simulink model "Circuit3_v3"  (R2020b)
settings: Solver=ode4  StartTime=0.0  StopTime=SIMTIME  FixedStep=step  RelTol=1e-3
values from neighbouring files (symbols this model uses):
  Be1 = 1300e6    (= 1300000000)    [Circut3_values.m]
  Be_p = 1300e6    (= 1300000000)    [Circut3_values.m]
  BeA = 1200e6    (= 1200000000)    [Circuit2_values.m]    (also in Circut3_values.m = 1300000000)
  BeB = 1500e6    (= 1500000000)    [Circuit2_values.m]    (also in Circut3_values.m = 1300000000)
  C_cv = (70/60000)/sqrt(5e5)    [Circut3_values.m]
  C_o = (1/60000)/sqrt(5e5)    [Circut3_values.m]
  C_v_valve = 1.16e-8    (= 1.16e-08)    [Circut3_values.m]
  g = 9.81    [Circut3_values.m]
  Jm = 3.6e-3    (= 0.0036)    [Circut3_values.m]
  Kp = (1.e-3)/(10e5)    (= 1e-09)    [Circuit1_load.m]    (also in Circuit2_values.m; Circut3_values.m)
  ml = 500    [Circut3_values.m]
  mw = 100    [Circut3_values.m]
  nm = 0.93    [Circut3_values.m]
  p0 = 1.e5    (= 100000)    [Circuit1_load.m]    (also in Circut3_values.m = 200000)
  p10 = 73e5    (= 7300000)    [Circut3_values.m]
  pA0 = 1e5    (= 100000)    [Circuit2_values.m]    (also in Circut3_values.m = 7300000)
  pB0 = 1e5    (= 100000)    [Circuit2_values.m]    (also in Circut3_values.m = 700000)
  pref = 180e5    (= 18000000)    [Circuit1_load.m]    (also in Circuit2_values.m; Circut3_values.m = 17000000)
  rho = 860    [Circuit1_load.m]    (also in Circuit2_values.m; Circut3_values.m)
  rw = 100e-3/2    (= 0.05)    [Circut3_values.m]
  tau_pump = 500e-3    (= 0.5)    [Circut3_values.m]
  tau_valve = 1.59e-2    (= 0.0159)    [Circut3_values.m]
  U_db = 2    [Circut3_values.m]
  V1 = 3e-3/2    (= 0.0015)    [Circut3_values.m]
  V_p = 3e-3    (= 0.003)    [Circut3_values.m]
  VA = 5e-4    (= 0.0005)    [Circuit2_values.m]    (also in Circut3_values.m = 0.0015)
  VB = 5e-4    (= 0.0005)    [Circuit2_values.m]    (also in Circut3_values.m = 0.003)
  Vm = 250e-6    (= 0.00025)    [Circut3_values.m]
undefined symbols (not defined in the file or in its folder): sigbuilder_block
settings Model: Creator=Janne  LastModifiedBy=Alex
settings DataIOCC: ReturnWorkspaceOutputs=off
settings DebuggingCC: ArithmeticOperatorsInVariantConditions=warning
settings SFSimCC: CustomCodeUndefinedFunction=UseInterfaceOnly

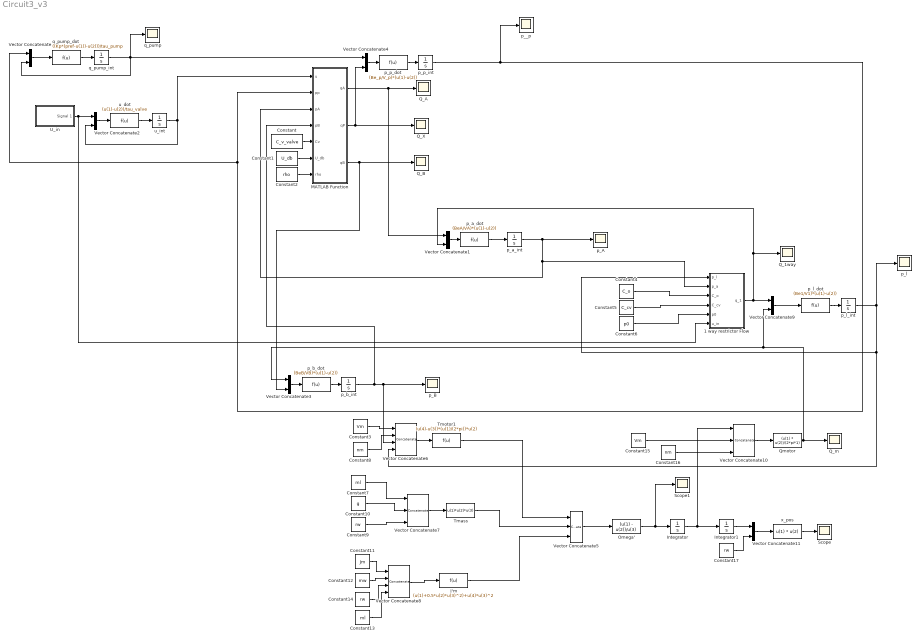
== system Circuit3_v3 ==
  1 way restrictor Flow : MATLAB Function  TreatAsAtomicUnit=on
  Constant : Constant  Value=C_v_valve
  Constant1 : Constant  Value=U_db
  Constant10 : Constant  Value=g
  Constant11 : Constant  Value=Jm
  Constant12 : Constant  Value=mw
  Constant13 : Constant  Value=ml
  Constant14 : Constant  Value=rw
  Constant15 : Constant  Value=Vm
  Constant16 : Constant  Value=nm
  Constant17 : Constant  Value=rw
  Constant2 : Constant  Value=rho
  Constant3 : Constant  Value=Vm
  Constant4 : Constant  Value=C_o
  Constant5 : Constant  Value=C_cv
  Constant6 : Constant  Value=p0
  Constant7 : Constant  Value=ml
  Constant8 : Constant  Value=nm
  Constant9 : Constant  Value=rw
  Integrator : Integrator
  Integrator1 : Integrator
  J'm : Fcn  Expr=(u(1)+0.5*u(2)*u(3)^2)+u(4)*u(3)^2
  MATLAB Function : MATLAB Function  TreatAsAtomicUnit=on
  Omega' : Fcn  Expr=(u(1) - u(2))/u(3)
  Q_1way : Scope
  Q_A : Scope
  Q_B : Scope
  Q_X : Scope
  Q_m : Scope
  Qmotor : Fcn  Expr=(u(1) * u(2))/(2*pi*1)
  Scope : Scope
  Scope1 : Scope
  Tmass : Fcn  Expr=u(1)*u(2)*u(3)
  Tmotor1 : Fcn  Expr=(u(4)-u(3))*(u(1)/(2*pi))*u(2)
  U_in : Subsystem  Tag=STV Subsys  LoadFcn=sigbuilder_block('load');  StartFcn=sigbuilder_block('start');  StopFcn=sigbuilder_block('stop');  ClipboardFcn=sigbuilder_block('clipboard');  mask(Sigbuilder block){tuvar=[0:10]}
      mask help: Simulink:masks:SigbuilderBlock_MD
      mask init:
      | if ~strcmp(get_param(bdroot(gcbh),'SimulationStatus'),'stopped') tuvar = sigbuilder_block('maskInit'); end
      settings: CopyFcn=sigbuilder_block('copy');  DeleteFcn=sigbuilder_block('delete');  ModelCloseFcn=sigbuilder_block('modelClose');  PreSaveFcn=sigbuilder_block('preSave');  PauseFcn=sigbuilder_block('pause');  ContinueFcn=sigbuilder_block('continue');  NameChangeFcn=sigbuilder_block('namechange');  OpenFcn=sigbuilder_block('open',[24.75 201.75 1008.75 309 ]);  CloseFcn=sigbuilder_block('close');
      mask Display: plot(0, 0, 100, 100,[2, 2, 32, 32, 2], [68, 8, 8, 68, 68],[32, 2], [38, 38], [32, 19, 2],[53, 60, 44], [32, 17, 17, 2],[16, 16, 31, 31]);txt = getActiveGroup(gcbh);text(2, 100, txt,'verticalAlignment', 'top');
  Vector Concatenate{,1..4,9,11} (7 alike) : Concatenate
  Vector Concatenate10 : Concatenate  NumInputs=3
  Vector Concatenate5 : Concatenate  NumInputs=3
  Vector Concatenate6 : Concatenate  NumInputs=4
  Vector Concatenate7 : Concatenate  NumInputs=3
  Vector Concatenate8 : Concatenate  NumInputs=4
  p_A : Scope
  p_B : Scope
  p__p : Scope
  p_a_dot : Fcn  Expr=(BeA/VA)*(u(1)-u(2))
  p_a_int : Integrator  InitialCondition=pA0  LimitOutput=on  UpperSaturationLimit=1000e5  LowerSaturationLimit=0
  p_b_dot : Fcn  Expr=(BeB/VB)*(u(1)-u(2))
  p_b_int : Integrator  InitialCondition=pB0  LimitOutput=on  UpperSaturationLimit=1000e5  LowerSaturationLimit=0
  p_l : Scope
  p_l_dot : Fcn  Expr=(Be1/V1)*(u(1)-u(2))
  p_l_int : Integrator  InitialCondition=p10  LimitOutput=on  UpperSaturationLimit=1000e5  LowerSaturationLimit=0
  p_p_dot : Fcn  Expr=(Be_p/V_p)*(u(1)-u(2))
  p_p_int : Integrator  LimitOutput=on  UpperSaturationLimit=1000e5  LowerSaturationLimit=0
  q_pump : Scope
  q_pump_dot : Fcn  Expr=((Kp*(pref-u(1))-u(2)))/tau_pump
  q_pump_int : Integrator  LimitOutput=on  UpperSaturationLimit=1000e5  LowerSaturationLimit=0
  u_dot : Fcn  Expr=(u(1)-u(2))/tau_valve
  u_int : Integrator  LimitOutput=on  UpperSaturationLimit=10  LowerSaturationLimit=-10
  x_pos : Fcn  Expr=u(1) * u(2)
  wires:
  q_pump_dot/1 -> q_pump_int/1
  Vector Concatenate/1 -> q_pump_dot/1
  q_pump_int/1 -> q_pump/1, Vector Concatenate/2, Vector Concatenate4/1
  Vector Concatenate4/1 -> p_p_dot/1
  p_p_dot/1 -> p_p_int/1
  p_p_int/1 -> Vector Concatenate/1, MATLAB Function/2(pp), p__p/1
  Constant/1 -> MATLAB Function/5(Cv)
  Constant1/1 -> MATLAB Function/6(U_db)
  Constant2/1 -> MATLAB Function/7(rho)
  p_a_dot/1 -> p_a_int/1
  p_b_dot/1 -> p_b_int/1
  Vector Concatenate1/1 -> p_a_dot/1
  Vector Concatenate3/1 -> p_b_dot/1
  p_a_int/1 -> 1 way restrictor Flow/2(p_a), MATLAB Function/3(pA), p_A/1
  MATLAB Function/1(qA) -> Vector Concatenate1/1, Q_A/1
  p_b_int/1 -> MATLAB Function/4(pB), Vector Concatenate6/3, p_B/1
  MATLAB Function/2(qP) -> Q_X/1, Vector Concatenate4/2
  MATLAB Function/3(qB) -> Vector Concatenate3/2, Q_B/1
  Constant6/1 -> 1 way restrictor Flow/5(p0)
  Constant5/1 -> 1 way restrictor Flow/4(C_cv)
  Constant4/1 -> 1 way restrictor Flow/3(C_o)
  u_int/1 -> Vector Concatenate2/2, MATLAB Function/1(u)
  Vector Concatenate2/1 -> u_dot/1
  u_dot/1 -> u_int/1
  U_in/1(Signal 1) -> 1 way restrictor Flow/6(u_in), Vector Concatenate2/1
  Vector Concatenate5/1 -> Omega'/1
  Constant3/1 -> Vector Concatenate6/1
  Constant8/1 -> Vector Concatenate6/2
  Vector Concatenate6/1 -> Tmotor1/1
  Constant7/1 -> Vector Concatenate7/1
  Constant10/1 -> Vector Concatenate7/2
  Constant9/1 -> Vector Concatenate7/3
  Vector Concatenate7/1 -> Tmass/1
  Constant11/1 -> Vector Concatenate8/1
  Constant12/1 -> Vector Concatenate8/2
  Constant14/1 -> Vector Concatenate8/3
  Constant13/1 -> Vector Concatenate8/4
  Tmotor1/1 -> Vector Concatenate5/1
  Tmass/1 -> Vector Concatenate5/2
  J'm/1 -> Vector Concatenate5/3
  Vector Concatenate8/1 -> J'm/1
  Omega'/1 -> Scope1/1, Integrator/1
  Integrator/1 -> Vector Concatenate10/1, Integrator1/1
  p_l_dot/1 -> p_l_int/1
  1 way restrictor Flow/1(q_1) -> Vector Concatenate9/1, Vector Concatenate1/2, Q_1way/1
  p_l_int/1 -> p_l/1, 1 way restrictor Flow/1(p_l), Vector Concatenate6/4
  Vector Concatenate9/1 -> p_l_dot/1
  Vector Concatenate10/1 -> Qmotor/1
  Constant15/1 -> Vector Concatenate10/2
  Constant16/1 -> Vector Concatenate10/3
  Qmotor/1 -> Vector Concatenate9/2, Vector Concatenate3/1, Q_m/1
  Integrator1/1 -> Vector Concatenate11/1
  Vector Concatenate11/1 -> x_pos/1
  x_pos/1 -> Scope/1
  Constant17/1 -> Vector Concatenate11/2

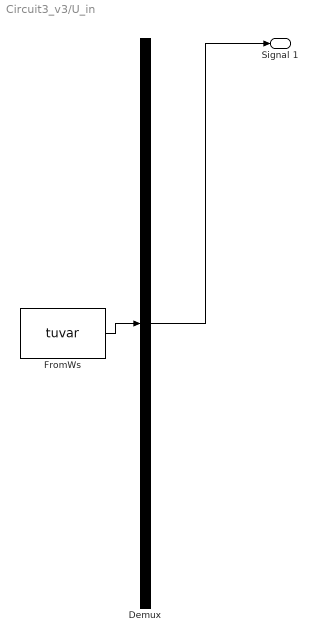
== system Circuit3_v3/U_in ==
  Demux : Demux  Tag=STV Demux  Outputs=1
      settings: DisplayOption=none
  FromWs : FromWorkspace  Tag=STV FromWs  VariableName=tuvar
      SigBuilderData=|
      | common.afterFinalStr = 'Extrapolate'
      | common.sampleTime = 0
      | dataSet.timeRange = [0 15]
      | dataSet.name = 'Group 1'
      | sbobj.Groups.Name = 'Group 1'
      | sbobj.Groups.Signals.Name = 'Signal 1'
      | sbobj.Groups.Signals.XData = [0 5.02 5.02 10 10 15]
      | sbobj.Groups.Signals.YData = [-10 -10 10 10 -10 -10]
      | sbobj.Groups.TimeRange = [0 15]
  Signal 1 : Outport  Tag=STV Outport
  wires:
  Demux/1 -> Signal 1/1
  FromWs/1 -> Demux/1

== matlab function Circuit3_v3/1 way restrictor Flow ==
  data: p_l input; p_a input; q_1 output; C_o input; C_cv input; p0 input; u_in input
function q_1  = fcn(p_l,p_a, C_o, C_cv, p0, u_in)
if u_in >= 0 && p_l - p_a >= p0
    C = C_cv;
else
    C = C_o;
end
q_1 = C*sqrt(abs(p_l - p_a))*sign(u_in);

== matlab function Circuit3_v3/MATLAB Function ==
  data: u input; pp input; pA input; pB input; qA output; Cv input; U_db input; rho input; qP output; qB output
function [qA,qP,qB] = fcn(u, pp, pA, pB, Cv, U_db, rho)

 if u >= (U_db)
    qA = Cv*u*sqrt(2*abs(pp-pA)/rho)*sign(pp-pA);

    qB = Cv*u*sqrt(2*pB/rho);

    qP = qA;
 elseif (u < U_db) 
    qB = Cv*u*sqrt(2*abs(pp-pB)/rho)*sign(pp-pB);

    qA = Cv*u*sqrt(2*pA/rho);

    qP = -qB;
 else 
    qA = 0;

    qB = 0;

    qP = 0;
 end
